simulink model "BrowarModel"  (R2024a)
settings: Solver=ode5  StartTime=0.0  StopTime=inf  FixedStep=0.1  RelTol=1e-3
undefined symbols (not defined in the file or in its folder): localhost, Matrikon, OI
libraries: opclib x24
(part 5 of 9)

== system BrowarModel/Kadz warzelna/Kadz warzelna/Model akumulacji ciepla w zbiorniku z ciecza ==
  Objetosc cieczy w zbiorniku : Inport
  Strumien odplywu cieczy : Inport  Port=2
  Strumien doplywu cieczy : Inport  Port=3
  Strumien cieplna dostepny : Inport  Port=4
  Strumien cieplo traconego : Inport  Port=5
  Temperatura strumien doplywu cieczy : Inport  Port=6
  1/gestosc cieczy : Gain  Gain=1/1000
  Cieplo : Integrator  LimitOutput=on  LowerSaturationLimit=0
  Cieplo parowania : Constant  Value=2257000
  Cieplo strumienia cieczy doplywajacej : Subsystem
  Cieplo strumienia cieczy odplywajacej : Subsystem
  "Cieplo wlasciwe " : Constant  Value=4189.9
  Display{,1..8} (9 alike) : Display
  Divide : Product  Inputs=/*
  Divide1 : Product  Inputs=*/
  Divide2 : Product  Inputs=*/
  "Dot " : DotProduct  OutDataTypeStr=Inherit: Inherit via internal rule
  Dot 1 : DotProduct  OutDataTypeStr=Inherit: Inherit via internal rule
  Gestosc cieczy : Gain  Gain=1000
  Saturation : Saturate  UpperLimit=inf  LowerLimit=0
  Sum{1..2,4..5} (4 alike) : Sum  Inputs=|+-
  Sum10 : Sum  Inputs=|++
  Sum3 : Sum  Inputs=|-+
  Sum7 : Sum  Inputs=|++
  Temperatura parowania : Constant  Value=100
  Zamiana C->K : Constant  Value=273.6
  Srumien cieczy odparowanej : Outport
  Srednia temperaturacie czy : Outport  Port=2
  Strumien ciepla odebrany : Outport  Port=3
  wires:
  Strumien cieplna dostepny/1 -> Strumien ciepla odebrany/1, Sum10/2  "J/s"
  Sum5/1 -> Sum4/1, Srednia temperaturacie czy/1, Display3/1
  Strumien doplywu cieczy/1 -> Cieplo strumienia cieczy doplywajacej/2(Strumien cieczy), Display6/1  "m3/s"
  Zamiana C->K/1 -> Sum5/2
  "Cieplo wlasciwe "/1 -> Divide1/2, Dot 1/2  "J/(kg*K)"
  Cieplo strumienia cieczy doplywajacej/1(Strumien ciepla) -> Sum3/2, Display1/1  "J/s"
  Temperatura strumien doplywu cieczy/1 -> Cieplo strumienia cieczy doplywajacej/1(Temperatura strumienia cieczy), Display8/1  "dec C"
  Divide1/1 -> Sum5/1, Cieplo strumienia cieczy odplywajacej/1(Temperatura strumienia cieczy)  "dec K"
  Divide/1 -> Divide1/1
  Cieplo/1 -> Divide/2, Display2/1  "J"
  Sum3/1 -> Sum1/1  "J/s"
  Strumien cieplo traconego/1 -> Sum1/2, Display7/1  "J/s"
  Sum1/1 -> Sum10/1  "J/s"
  Sum10/1 -> Sum2/1  "J/s"
  Temperatura parowania/1 -> Sum4/2  "dec C"
  Sum4/1 -> Saturation/1
  Saturation/1 -> Dot 1/1
  Dot 1/1 -> "Dot "/1
  "Dot "/1 -> Divide2/1, Sum2/2  "J/s"
  Sum2/1 -> Cieplo/1  "J/s"
  Cieplo strumienia cieczy odplywajacej/1(Strumien ciepla) -> Sum3/1, Display/1  "J/s"
  1/gestosc cieczy/1 -> Sum7/2, Srumien cieczy odparowanej/1  "m3/s"
  Divide2/1 -> 1/gestosc cieczy/1  "kg/s"
  Cieplo parowania/1 -> Divide2/2  "J/kg"
  Objetosc cieczy w zbiorniku/1 -> Gestosc cieczy/1  "m3"
  Gestosc cieczy/1 -> "Dot "/2, Divide/1, Display4/1  "kg"
  Sum7/1 -> Cieplo strumienia cieczy odplywajacej/2(Strumien cieczy)
  Strumien odplywu cieczy/1 -> Sum7/1, Display5/1  "m3/s"

== system BrowarModel/Kadz warzelna/Kadz warzelna/Model jakosci brzeczki wejsciowej ==
  note: Model jakosci brzeczki w zbiorniku
  Objetosc : Inport
  Przepelnienie : Inport  Port=2
  Doplyw brzeczki : Inport  Port=3
  Odplyw : Inport  Port=4
  Jakosc brzeczki : Inport  Port=5
  Divide1 : Product  Inputs=/*
  Jakosc brzeczki x objetosc : Integrator  LimitOutput=on  LowerSaturationLimit=0
  Product3 : Product  RndMeth=Zero
  Product4 : Product  RndMeth=Zero
  Product6 : Product  RndMeth=Zero
  Relational Operator : RelationalOperator  Operator=<  InputSameDT=off
  Sat : Constant
  Sum5 : Sum  Inputs=|+-
  Jakosc brzeczki zbiornika : Outport
  wires:
  Sum5/1 -> Jakosc brzeczki x objetosc/1
  Product4/1 -> Product3/2
  Sat/1 -> Relational Operator/2
  Jakosc brzeczki x objetosc/1 -> Divide1/2
  Divide1/1 -> Product6/1, Jakosc brzeczki zbiornika/1
  Product3/1 -> Sum5/1
  Relational Operator/1 -> Product3/1
  Product6/1 -> Sum5/2
  Objetosc/1 -> Divide1/1
  Doplyw brzeczki/1 -> Product4/1
  Odplyw/1 -> Product6/2
  Przepelnienie/1 -> Relational Operator/1
  Jakosc brzeczki/1 -> Product4/2

== system BrowarModel/Kadz warzelna/Kadz warzelna/Model jakosci warzenia ==
  note: Model jakosci warzenia
  Srednia temperatura : Inport
  Odplyw : Inport  Port=2
  Doplyw brzeczki : Inport  Port=3
  Doplyw chmielu : Inport  Port=4
  Constant : Constant  Value=48
  Display : Display
  Display1 : Display
  Divide : Product  Inputs=*/
  Divide1 : Product  Inputs=/*
  "Gotowanie " : Subsystem
  Jakosc mieszaniny : Lookup  InputValues=[0 0.001 0.00175 0.001875 0.002 0.002125 0.00225 0.003 0.005 0.0075]  Table=[0 0.2 0.5 1 1 1 0.5 0.2 0 0]  SaturateOnIntegerOverflow=off
  Objetosc brzeczka : Integrator  InitialCondition=0.001  LimitOutput=on  UpperSaturationLimit=48  LowerSaturationLimit=0.001
  Objetosc chmiel : Integrator  LimitOutput=on  UpperSaturationLimit=48  LowerSaturationLimit=0
  Odplyw brzeczka : DotProduct  OutDataTypeStr=Inherit: Inherit via internal rule
  Odplyw chmielu : DotProduct  OutDataTypeStr=Inherit: Inherit via internal rule
  Przepelnienie - brzeczka : DotProduct  OutDataTypeStr=Inherit: Inherit via internal rule
  Przepelnienie - chmiel : DotProduct  OutDataTypeStr=Inherit: Inherit via internal rule
  Relational Operator : RelationalOperator  Operator=<  InputSameDT=off
  Saturation : Saturate  UpperLimit=inf  LowerLimit=0
  Sum5 : Sum  Inputs=-+
  Sum6 : Sum  Inputs=+-
  Sum7 : Sum
  Jakosc : Outport
  wires:
  Sum6/1 -> Objetosc brzeczka/1
  Odplyw brzeczka/1 -> Sum6/2
  Objetosc chmiel/1 -> Sum7/1, Divide/1
  Objetosc brzeczka/1 -> Sum7/2, Divide1/2
  Sum7/1 -> Divide1/1, Divide/2, Relational Operator/1, "Gotowanie "/3(Objetosc mieszaniny)  "m3"
  Odplyw chmielu/1 -> Sum5/1
  Divide/1 -> Odplyw chmielu/1, Jakosc mieszaniny/1
  Divide1/1 -> Odplyw brzeczka/2
  Sum5/1 -> Objetosc chmiel/1
  Przepelnienie - chmiel/1 -> Sum5/2
  Przepelnienie - brzeczka/1 -> Sum6/1
  Relational Operator/1 -> Przepelnienie - chmiel/2, Przepelnienie - brzeczka/1
  Constant/1 -> Relational Operator/2
  Odplyw/1 -> Odplyw brzeczka/1, "Gotowanie "/4(Odplyw), Odplyw chmielu/2  "m3/s"
  "Gotowanie "/1(Jakosc) -> Saturation/1, Display1/1
  Jakosc mieszaniny/1 -> "Gotowanie "/2(Jakosc mieszaniny), Display/1  "[0,1]"
  Saturation/1 -> Jakosc/1
  Srednia temperatura/1 -> "Gotowanie "/1(Srednia temperatura)  "decC"
  Doplyw chmielu/1 -> Przepelnienie - chmiel/1  "m3/s"
  Doplyw brzeczki/1 -> Przepelnienie - brzeczka/2  "m3/s"

== system BrowarModel/Kadz warzelna/Kadz warzelna/Model ogrzewacza ==
  note: Ogrzewacz elektryczny
  note: Uszkodzenie ogrzewacza
  Sterowanie : Inport
  Spadek mocy : Inport  Port=2
  Booster : Product  RndMeth=Zero
  "Booster " : Subsystem
  Booster block : Subsystem
  Const : Constant  Value=100
  GUIMon : Gain
  Gain : Gain  Gain=1/100
  Gain1 : Gain  Gain=1/100
  Maksymalna moc : Constant  Value=10000000
  Product : Product  RndMeth=Zero
  Product1 : Product  RndMeth=Zero
  Quantizer : Quantizer  QuantizationInterval=20
  Sat ster : Saturate  UpperLimit=100  LowerLimit=0
  Sat uszk : Saturate  UpperLimit=100  LowerLimit=0
  Sat zero : Saturate  UpperLimit=inf  LowerLimit=0
  Sum1 : Sum  Inputs=|+-
  Sum2 : Sum  Inputs=|+-
  Transfer Fcn : TransferFcn  Denominator=[30 1]
  Transfer Fcn1 : TransferFcn  Denominator=[30 1]
  Zaklocenia : Subsystem
  Cieplo dostarczone : Outport
  wires:
  Sat ster/1 -> Quantizer/1
  Sterowanie/1 -> Sat ster/1
  Quantizer/1 -> GUIMon/1
  Gain/1 -> Product/1
  Zaklocenia/1(Out) -> Sum1/2
  Product/1 -> Transfer Fcn/1
  Transfer Fcn/1 -> Transfer Fcn1/1, "Booster "/1(In1)
  Sum1/1 -> Sat zero/1
  GUIMon/1 -> Gain/1
  Sat zero/1 -> Cieplo dostarczone/1
  Maksymalna moc/1 -> Product1/1
  Spadek mocy/1 -> Sat uszk/1
  Sat uszk/1 -> Sum2/2
  Sum2/1 -> Gain1/1
  Const/1 -> Sum2/1
  Gain1/1 -> Product1/2
  Product1/1 -> Booster/1
  Booster block/1(Out) -> Booster/2
  Booster/1 -> Product/2
  "Booster "/1(Out) -> Zaklocenia/1(In), Sum1/1
  Transfer Fcn1/1 -> "Booster "/2(In2)

== system BrowarModel/Kadz warzelna/Kadz warzelna/Model rozkladu temperatur ==
  Poziom : Inport
  Srednia temperatura : Inport  Port=2
  " Dot 1" : DotProduct  OutDataTypeStr=Inherit: Inherit via internal rule
  " Dot 2" : DotProduct  OutDataTypeStr=Inherit: Inherit via internal rule
  " Dot 3" : DotProduct  OutDataTypeStr=Inherit: Inherit via internal rule
  Divide2 : Product  Inputs=/*
  Divide3 : Product  Inputs=/*
  Divide4 : Product  Inputs=/*
  Model rozkladu temperatur : Subsystem
  Pozycja sensor dolny : Constant  Value=0.5
  Pozycja sensor gorny : Constant  Value=2.5
  Pozycja sensor srodkowy : Constant  Value=1.5
  Sensor dolny niezanuzony : RelationalOperator  Operator=<  InputSameDT=off
  Sensor gorny niezanuzony : RelationalOperator  Operator=<  InputSameDT=off
  Sensor srodkowy niezanuzony : RelationalOperator  Operator=<  InputSameDT=off
  Sum13 : Sum  Inputs=|+-
  Sum14 : Sum  Inputs=|+-
  Sum15 : Sum  Inputs=|+-
  Switch : Switch  Threshold=0.5  SaturateOnIntegerOverflow=off  InputSameDT=off
  Switch1 : Switch  Threshold=0.5  SaturateOnIntegerOverflow=off  InputSameDT=off
  Switch2 : Switch  Threshold=0.5  SaturateOnIntegerOverflow=off  InputSameDT=off
  "Temperatura pokojowa (deg C) " : Constant  Value=22
  Temperatura lustra zbiornika : Outport
  Sensor temperatury gorny : Outport  Port=2
  Sensor temperatury srodkowy : Outport  Port=3
  Sensor temperatury dolny : Outport  Port=4
  Temperatura przy dnie zbiornika : Outport  Port=5
  wires:
  Model rozkladu temperatur/1(Temperatura przy powierzchni) -> Temperatura lustra zbiornika/1
  Poziom/1 -> Divide4/1, Divide3/1, Divide2/1, Sensor dolny niezanuzony/1, Sensor srodkowy niezanuzony/1, Sensor gorny niezanuzony/1, Model rozkladu temperatur/1(Poziom)  "m"
  Switch2/1 -> Sensor temperatury dolny/1
  Switch/1 -> Sensor temperatury gorny/1
  " Dot 3"/1 -> Sum15/2
  Divide2/1 -> " Dot 3"/2
  Divide3/1 -> " Dot 2"/2
  " Dot 2"/1 -> Sum14/2
  " Dot 1"/1 -> Sum13/2
  Divide4/1 -> " Dot 1"/2
  Model rozkladu temperatur/2(Temperatura przy dnie) -> Sum15/1, Sum14/1, Sum13/1, Temperatura przy dnie zbiornika/1
  Sum15/1 -> Switch2/3
  Sum14/1 -> Switch1/3
  Sum13/1 -> Switch/3
  Switch1/1 -> Sensor temperatury srodkowy/1
  Sensor dolny niezanuzony/1 -> Switch2/2
  Sensor srodkowy niezanuzony/1 -> Switch1/2
  Sensor gorny niezanuzony/1 -> Switch/2
  Pozycja sensor dolny/1 -> Divide2/2, Sensor dolny niezanuzony/2
  Pozycja sensor srodkowy/1 -> Divide3/2, Sensor srodkowy niezanuzony/2
  Pozycja sensor gorny/1 -> Divide4/2, Sensor gorny niezanuzony/2
  "Temperatura pokojowa (deg C) "/1 -> Switch2/1, Switch1/1, Switch/1, Model rozkladu temperatur/2(Temperatura otoczenia)
  Model rozkladu temperatur/3(Gradient temperatury) -> " Dot 1"/1, " Dot 2"/1, " Dot 3"/1
  Srednia temperatura/1 -> Model rozkladu temperatur/3(Srednia temperatura)  "decC"

== system BrowarModel/Kadz warzelna/Kadz warzelna/Model utratu ciepla ==
  Poziom : Inport
  Pole podstawy zbiornika : Inport  Port=2
  Srednia temperatura : Inport  Port=3
  Temperatura lustra : Inport  Port=4
  Cieplo tracone przez pow. gorna : DotProduct  OutDataTypeStr=Inherit: Inherit via internal rule
  Cieplo tracone przez scianki : DotProduct  OutDataTypeStr=Inherit: Inherit via internal rule
  Pow ->obwod : Fcn  Expr=2*3.14*sqrt(u(1)/3.14)
  Pow styku scian bocznych : DotProduct  OutDataTypeStr=Inherit: Inherit via internal rule
  Saturation : Saturate  UpperLimit=inf  LowerLimit=0
  Sum11 : Sum  Inputs=|-+
  Sum12 : Sum  Inputs=|-+
  Sum2 : Sum
  "Temperatura pokojowa (deg C)  " : Constant  Value=22
  Wspolczynnik przenikania ciepla : Gain  Gain=950
  Wspolczynnik przenikania ciepla scian : Gain  Gain=450
  Strumien ciepla : Outport
  wires:
  Temperatura lustra/1 -> Sum12/2  "dec C"
  Sum2/1 -> Saturation/1
  Srednia temperatura/1 -> Sum11/2  "dec C"
  Pole podstawy zbiornika/1 -> Wspolczynnik przenikania ciepla/1, Pow ->obwod/1
  Poziom/1 -> Pow styku scian bocznych/1
  Sum11/1 -> Cieplo tracone przez scianki/2
  "Temperatura pokojowa (deg C)  "/1 -> Sum12/1, Sum11/1
  Cieplo tracone przez pow. gorna/1 -> Sum2/2
  Cieplo tracone przez scianki/1 -> Sum2/1
  Wspolczynnik przenikania ciepla scian/1 -> Cieplo tracone przez scianki/1
  Pow styku scian bocznych/1 -> Wspolczynnik przenikania ciepla scian/1  "m2"
  Pow ->obwod/1 -> Pow styku scian bocznych/2
  Sum12/1 -> Cieplo tracone przez pow. gorna/1
  Wspolczynnik przenikania ciepla/1 -> Cieplo tracone przez pow. gorna/2
  Saturation/1 -> Strumien ciepla/1  "J/s"

== system BrowarModel/Kadz warzelna/Kadz warzelna/Odplyw z kadzi ==
  note: Doplyw kadzi
  Sterowanie zaworu : Inport
  Przeciek zaworu : Inport  Port=2
  Dlawienie zaworu : Inport  Port=3
  Wyciek : Inport  Port=4
  Poziom w kadzi : Inport  Port=5
  Zalaczenie pompy : Inport  Port=6
  Sterowanie pompy : Inport  Port=7
  Uszkodzenie pompy : Inport  Port=8
  Charakterystyka pompy : Lookup  InputValues="[0\t125\t250\t375\t500\t625\t750\t875\t1000\t1125\t1250\t1375\t1500 1625]"  Table=|  SaturateOnIntegerOverflow=off
      | [0 50	125	178	220	250	270	288	300	310	315	320	323	327
      | ]
  Gain : Gain  Gain=1/100
  Obciazenie silnika : Gain  Gain=1/500
  Product : Product  RndMeth=Zero
  Product1 : Product  RndMeth=Zero
  Relay : Relay  OnOutputValue=0  OffOutputValue=1
  Relay1 : Relay
  Sat uszk : Saturate  UpperLimit=100  LowerLimit=0
  Silnik elektryczny : Subsystem
  "Sterowanie " : DotProduct  OutDataTypeStr=Inherit: Inherit via internal rule
  Straty pompy : Gain  Gain=50/0.15
  Sum : Sum  Inputs=|+-
  Sum1 : Sum  Inputs=|+-
  Wplyw stopnia wypelnienia kadzi : Lookup  InputValues=[-1, 0, 0.05, 1]  Table=[0, 0, 1,1]  SaturateOnIntegerOverflow=off
  Wplyw uszkodzenia : Product  RndMeth=Zero
  Zawor dyskretny : Subsystem
  Przeplyw_wyciek : Outport
  Przeplyw : Outport  Port=2
  Obroty : Outport  Port=3
  Prad silnika : Outport  Port=4
  Silnik Idle : Outport  Port=5
  Silnik Running : Outport  Port=6
  Silnik Alarm : Outport  Port=7
  wires:
  Wplyw stopnia wypelnienia kadzi/1 -> Product/1  "[0,1]"
  Zawor dyskretny/1(Przeplyw) -> Sum1/1, Straty pompy/1, Product1/1
  Dlawienie zaworu/1 -> Zawor dyskretny/4(Dlawienie)
  Poziom w kadzi/1 -> Wplyw stopnia wypelnienia kadzi/1  "m"
  Zalaczenie pompy/1 -> Relay1/1, Silnik elektryczny/1(Zalaczenie)
  Uszkodzenie pompy/1 -> Relay/1, Silnik elektryczny/4(Uszkodzenie)
  Relay/1 -> Wplyw uszkodzenia/2
  Silnik elektryczny/1(Obroty) -> Charakterystyka pompy/1, Obroty/1
  Wplyw uszkodzenia/1 -> Product/2
  Charakterystyka pompy/1 -> "Sterowanie "/2  "kPa"
  "Sterowanie "/1 -> Wplyw uszkodzenia/1
  Relay1/1 -> "Sterowanie "/1
  Product/1 -> Sum/1, Obciazenie silnika/1
  Sum/1 -> Zawor dyskretny/2(Cisnienie)
  Straty pompy/1 -> Sum/2
  Wyciek/1 -> Sat uszk/1
  Product1/1 -> Przeplyw_wyciek/1, Sum1/2
  Sum1/1 -> Przeplyw/1
  Sat uszk/1 -> Gain/1
  Przeciek zaworu/1 -> Zawor dyskretny/3(Przeciek)
  Sterowanie zaworu/1 -> Zawor dyskretny/1(Sterowanie)
  Gain/1 -> Product1/2
  Silnik elektryczny/2(Prad) -> Prad silnika/1
  Silnik elektryczny/3(Idle) -> Silnik Idle/1
  Silnik elektryczny/4(Running) -> Silnik Running/1
  Silnik elektryczny/5(Alarm) -> Silnik Alarm/1
  Sterowanie pompy/1 -> Silnik elektryczny/2(Zadane obroty)
  Obciazenie silnika/1 -> Silnik elektryczny/3(Obciazenie zew)

== system BrowarModel/Kadz warzelna/Kadz warzelna/Poziom zbiornika ==
  Objetosc : Inport
  Powierzchnia dna : Inport  Port=2
  1/powierzchnia : Product  Inputs=*/
  Pozycja sensora max (2.8 m) : Constant  Value=2.8
  Pozycja sensora min (0.2 m) : Constant  Value=.2
  Sensor max : RelationalOperator  InputSameDT=off
  Sensor min : RelationalOperator  InputSameDT=off
  Poziom  wysoki : Outport
  Poziom niski : Outport  Port=2
  Poziom : Outport  Port=3
  wires:
  Objetosc/1 -> 1/powierzchnia/1  "m3"
  Powierzchnia dna/1 -> 1/powierzchnia/2  "m2"
  Sensor min/1 -> Poziom niski/1
  Sensor max/1 -> Poziom  wysoki/1
  Pozycja sensora min (0.2 m)/1 -> Sensor min/2
  Pozycja sensora max (2.8 m)/1 -> Sensor max/2
  1/powierzchnia/1 -> Poziom/1, Sensor max/1, Sensor min/1  "m"

== system BrowarModel/Kadz warzelna/Kadz warzelna/Wyciek ==
  note: Kadz warzelna - wyciek
  Wyciek : Inport
  Poziom : Inport  Port=2
  Gain : Gain  Gain=1/3
  Math Function : Math  Operator=sqrt  SignedPower=on
  Max wyciek : Constant  Value=0.1
  Product : Product  RndMeth=Zero
  Product1 : Product  RndMeth=Zero
  Sat uszk (F>=0)1 : Saturate  UpperLimit=1  LowerLimit=0
  Strumien wycieku : Outport
  wires:
  Sat uszk (F>=0)1/1 -> Product/1
  Product1/1 -> Product/2
  Max wyciek/1 -> Product1/1  "m3/s"
  Math Function/1 -> Product1/2
  Gain/1 -> Math Function/1
  Poziom/1 -> Gain/1
  Wyciek/1 -> Sat uszk (F>=0)1/1
  Product/1 -> Strumien wycieku/1

== system BrowarModel/Kadz warzelna/LT401/Zaklocenia pomiarowe ==
  Product1 : Product  InputSameDT=on  RndMeth=Zero  SaturateOnIntegerOverflow=on  OutDataTypeStr=Inherit: Same as first input
  Product3 : Product  InputSameDT=on  RndMeth=Zero  SaturateOnIntegerOverflow=on  OutDataTypeStr=Inherit: Same as first input
  Random Number : RandomNumber  Variance=.5  Seed=4365624  SampleTime=0.1
  Transfer Fcn1 : TransferFcn  Denominator=[0.5 1]
  Transfer Fcn2 : TransferFcn  Denominator=[0.5 1]
  Zaklocenia pomiarowe : Constant  Value=ZakloceniaPom
  Out : Outport
  wires:
  Product1/1 -> Product3/2
  [ZaklPom] -> Product1/1
  Zaklocenia pomiarowe/1 -> Product1/2
  Transfer Fcn2/1 -> Out/1
  Transfer Fcn1/1 -> Transfer Fcn2/1
  Product3/1 -> Transfer Fcn1/1
  Random Number/1 -> Product3/1

== system BrowarModel/Kadz warzelna/ST404/Zaklocenia pomiarowe ==
  Product1 : Product  InputSameDT=on  RndMeth=Zero  SaturateOnIntegerOverflow=on  OutDataTypeStr=Inherit: Same as first input
  Product3 : Product  InputSameDT=on  RndMeth=Zero  SaturateOnIntegerOverflow=on  OutDataTypeStr=Inherit: Same as first input
  Random Number : RandomNumber  Variance=.5  Seed=4365624  SampleTime=0.1
  Transfer Fcn1 : TransferFcn  Denominator=[0.5 1]
  Transfer Fcn2 : TransferFcn  Denominator=[0.5 1]
  Zaklocenia pomiarowe : Constant  Value=ZakloceniaPom
  Out : Outport
  wires:
  Product1/1 -> Product3/2
  [ZaklPom] -> Product1/1
  Zaklocenia pomiarowe/1 -> Product1/2
  Transfer Fcn2/1 -> Out/1
  Transfer Fcn1/1 -> Transfer Fcn2/1
  Product3/1 -> Transfer Fcn1/1
  Random Number/1 -> Product3/1

== system BrowarModel/Kadz warzelna/TT402H/Zaklocenia pomiarowe ==
  Product1 : Product  InputSameDT=on  RndMeth=Zero  SaturateOnIntegerOverflow=on  OutDataTypeStr=Inherit: Same as first input
  Product3 : Product  InputSameDT=on  RndMeth=Zero  SaturateOnIntegerOverflow=on  OutDataTypeStr=Inherit: Same as first input
  Random Number : RandomNumber  Variance=.5  Seed=4365624  SampleTime=0.1
  Transfer Fcn1 : TransferFcn  Denominator=[0.5 1]
  Transfer Fcn2 : TransferFcn  Denominator=[0.5 1]
  Zaklocenia pomiarowe : Constant  Value=ZakloceniaPom
  Out : Outport
  wires:
  Random Number/1 -> Product3/1
  Product3/1 -> Transfer Fcn1/1
  Transfer Fcn1/1 -> Transfer Fcn2/1
  Transfer Fcn2/1 -> Out/1
  Zaklocenia pomiarowe/1 -> Product1/2
  [ZaklPom] -> Product1/1
  Product1/1 -> Product3/2

== system BrowarModel/Kadz warzelna/TT402L/Zaklocenia pomiarowe ==
  Product1 : Product  InputSameDT=on  RndMeth=Zero  SaturateOnIntegerOverflow=on  OutDataTypeStr=Inherit: Same as first input
  Product3 : Product  InputSameDT=on  RndMeth=Zero  SaturateOnIntegerOverflow=on  OutDataTypeStr=Inherit: Same as first input
  Random Number : RandomNumber  Variance=.5  Seed=4365624  SampleTime=0.1
  Transfer Fcn1 : TransferFcn  Denominator=[0.5 1]
  Transfer Fcn2 : TransferFcn  Denominator=[0.5 1]
  Zaklocenia pomiarowe : Constant  Value=ZakloceniaPom
  Out : Outport
  wires:
  Random Number/1 -> Product3/1
  Product3/1 -> Transfer Fcn1/1
  Transfer Fcn1/1 -> Transfer Fcn2/1
  Transfer Fcn2/1 -> Out/1
  Zaklocenia pomiarowe/1 -> Product1/2
  [ZaklPom] -> Product1/1
  Product1/1 -> Product3/2

== system BrowarModel/Kadz warzelna/TT402M/Zaklocenia pomiarowe ==
  Product1 : Product  InputSameDT=on  RndMeth=Zero  SaturateOnIntegerOverflow=on  OutDataTypeStr=Inherit: Same as first input
  Product3 : Product  InputSameDT=on  RndMeth=Zero  SaturateOnIntegerOverflow=on  OutDataTypeStr=Inherit: Same as first input
  Random Number : RandomNumber  Variance=.5  Seed=4365624  SampleTime=0.1
  Transfer Fcn1 : TransferFcn  Denominator=[0.5 1]
  Transfer Fcn2 : TransferFcn  Denominator=[0.5 1]
  Zaklocenia pomiarowe : Constant  Value=ZakloceniaPom
  Out : Outport
  wires:
  Product1/1 -> Product3/2
  [ZaklPom] -> Product1/1
  Zaklocenia pomiarowe/1 -> Product1/2
  Transfer Fcn2/1 -> Out/1
  Transfer Fcn1/1 -> Transfer Fcn2/1
  Product3/1 -> Transfer Fcn1/1
  Random Number/1 -> Product3/1

== system BrowarModel/Kadz zacierna/ET205/Zaklocenia pomiarowe ==
  Product1 : Product  InputSameDT=on  RndMeth=Zero  SaturateOnIntegerOverflow=on  OutDataTypeStr=Inherit: Same as first input
  Product3 : Product  InputSameDT=on  RndMeth=Zero  SaturateOnIntegerOverflow=on  OutDataTypeStr=Inherit: Same as first input
  Random Number : RandomNumber  Variance=.5  Seed=4365624  SampleTime=0.1
  Transfer Fcn1 : TransferFcn  Denominator=[0.5 1]
  Transfer Fcn2 : TransferFcn  Denominator=[0.5 1]
  Zaklocenia pomiarowe : Constant  Value=ZakloceniaPom
  Out : Outport
  wires:
  Random Number/1 -> Product3/1
  Product3/1 -> Transfer Fcn1/1
  Transfer Fcn1/1 -> Transfer Fcn2/1
  Transfer Fcn2/1 -> Out/1
  Zaklocenia pomiarowe/1 -> Product1/2
  [ZaklPom] -> Product1/1
  Product1/1 -> Product3/2

== system BrowarModel/Kadz zacierna/FT201/Zaklocenia pomiarowe ==
  Product1 : Product  InputSameDT=on  RndMeth=Zero  SaturateOnIntegerOverflow=on  OutDataTypeStr=Inherit: Same as first input
  Product3 : Product  InputSameDT=on  RndMeth=Zero  SaturateOnIntegerOverflow=on  OutDataTypeStr=Inherit: Same as first input
  Random Number : RandomNumber  Variance=.5  Seed=4365624  SampleTime=0.1
  Transfer Fcn1 : TransferFcn  Denominator=[0.5 1]
  Transfer Fcn2 : TransferFcn  Denominator=[0.5 1]
  Zaklocenia pomiarowe : Constant  Value=ZakloceniaPom
  Out : Outport
  wires:
  Random Number/1 -> Product3/1
  Product3/1 -> Transfer Fcn1/1
  Transfer Fcn1/1 -> Transfer Fcn2/1
  Transfer Fcn2/1 -> Out/1
  Zaklocenia pomiarowe/1 -> Product1/2
  [ZaklPom] -> Product1/1
  Product1/1 -> Product3/2

== system BrowarModel/Kadz zacierna/Kadz zacierna/Kadz zacierna ==
  note: Kadz
  Doplyw wody : Inport
  Temperatura doplywu wody : Inport  Port=2
  Doplyw sruty : Inport  Port=3
  Temperatura doplywu sruty : Inport  Port=4
  Odplyw : Inport  Port=5
  Dostepny strumien ciepla : Inport  Port=6
  Obroty mieszadla : Inport  Port=7
  Wyciek : Inport  Port=8
  Gain : Gain  Gain=1/1.5
  Math Function : Math  Operator=sqrt  SignedPower=on
  Max wyciek : Constant  Value=0.1
  Model akumulacji ciepla w zbiorniku z ciecza : Subsystem
  Model jakosci zacieru : Subsystem
  Model rozkladu temperatur : Subsystem
  Model utratu ciepla : Subsystem
  Objetosc : Integrator  InitialCondition=0.001  LimitOutput=on  UpperSaturationLimit=48  LowerSaturationLimit=0.001  ShowSaturationPort=on
  Powierzchnia dna m2 : Constant  Value=32
  Poziom zbiornika : Subsystem
  Product : Product  RndMeth=Zero
  Product1 : Product  RndMeth=Zero
  Sat doplyw (F>=0) : Saturate  UpperLimit=inf  LowerLimit=0
  Sat uszk (F>=0)1 : Saturate  UpperLimit=1  LowerLimit=0
  Saturation : Saturate  UpperLimit=inf  LowerLimit=0
  Sum1 : Sum  Inputs=|+-
  Sum2 : Sum  Inputs=|+-
  Sum3 : Sum  Inputs=|++
  Sum4 : Sum  Inputs=|++
  Poziom : Outport
  Poziom wysoki : Outport  Port=2
  Poziom niski : Outport  Port=3
  Temperatura sensor gorny : Outport  Port=4
  Temperatura sensor srodkowy : Outport  Port=5
  Temperatura sensor dolny : Outport  Port=6
  Temperatura dna : Outport  Port=7
  Jakosc zacieru : Outport  Port=8
  Temperatura srednia : Outport  Port=9
  wires:
  Temperatura doplywu wody/1 -> Model akumulacji ciepla w zbiorniku z ciecza/6(Temperatura strumien doplywu wody)
  Model akumulacji ciepla w zbiorniku z ciecza/1(Srumien cieczy odparowanej) -> Sum2/2  "m3/s"
  Sum1/1 -> Sum2/1
  Sum2/1 -> Objetosc/1
  Poziom zbiornika/3(Poziom) -> Poziom/1, Model utratu ciepla/1(Poziom), Model rozkladu temperatur/1(Poziom), Gain/1
  Objetosc/1 -> Poziom zbiornika/1(Objetosc), Model akumulacji ciepla w zbiorniku z ciecza/1(Objetosc cieczy w zbiorniku)  "m3"
  Poziom zbiornika/1(Poziom  wysoki) -> Poziom wysoki/1
  Poziom zbiornika/2(Poziom niski) -> Poziom niski/1
  Powierzchnia dna m2/1 -> Poziom zbiornika/2(Powierzchnia dna), Model utratu ciepla/2(Pole podstawy zbiornika)  "m2"
  Model akumulacji ciepla w zbiorniku z ciecza/2(Srednia temperaturacie czy) -> Model utratu ciepla/3(Srednia temperatura), Model rozkladu temperatur/2(Srednia temperatura), Model jakosci zacieru/1(Srednia temperatura), Temperatura srednia/1
  Model utratu ciepla/1(Strumien ciepla) -> Model akumulacji ciepla w zbiorniku z ciecza/9(Strumien cieplo traconego)
  Model rozkladu temperatur/1(Temperatura lustra zbiornika) -> Model utratu ciepla/4(Temperatura lustra)  "dec C"
  Doplyw sruty/1 -> Sat doplyw (F>=0)/1
  Model rozkladu temperatur/2(Sensor temperatury gorny) -> Temperatura sensor gorny/1
  Model rozkladu temperatur/3(Sensor temperatury srodkowy) -> Temperatura sensor srodkowy/1
  Model rozkladu temperatur/4(Sensor temperatury dolny) -> Temperatura sensor dolny/1
  Obroty mieszadla/1 -> Model rozkladu temperatur/3(Obroty mieszadla), Model jakosci zacieru/5(Obroty mieszadla)
  Dostepny strumien ciepla/1 -> Model akumulacji ciepla w zbiorniku z ciecza/8(Strumien cieplna dostepny)  "J/s"
  Model rozkladu temperatur/5(Temperatura przy dnie zbiornika) -> Temperatura dna/1
  Sat doplyw (F>=0)/1 -> Sum3/1, Model akumulacji ciepla w zbiorniku z ciecza/5(Strumien sruty), Model jakosci zacieru/4(Doplyw srutu)  "m3/s"
  Sum3/1 -> Sum1/1
  Doplyw wody/1 -> Sum3/2, Model akumulacji ciepla w zbiorniku z ciecza/4(Strumien doplywu wody), Model jakosci zacieru/3(Doplyw wody)  "m3/h"
  Temperatura doplywu sruty/1 -> Model akumulacji ciepla w zbiorniku z ciecza/7(Temperatura strumien doplywu sruty)
  Sum4/1 -> Model akumulacji ciepla w zbiorniku z ciecza/3(Strumien odplywu cieczy), Model jakosci zacieru/2(Odplyw), Sum1/2
  Odplyw/1 -> Saturation/1  "m3/h"
  Wyciek/1 -> Sat uszk (F>=0)1/1
  Product/1 -> Sum4/2
  Sat uszk (F>=0)1/1 -> Product/1
  Model jakosci zacieru/1(Jakosc) -> Jakosc zacieru/1
  Product1/1 -> Product/2
  Max wyciek/1 -> Product1/1  "m3/s"
  Math Function/1 -> Product1/2
  Gain/1 -> Math Function/1
  Objetosc/2 -> Model akumulacji ciepla w zbiorniku z ciecza/2(Przepelnienie)
  Saturation/1 -> Sum4/1

== system BrowarModel/Kadz zacierna/Kadz zacierna/Model mieszadla ==
  note: Model mieszadla
  note: Uszkodzenie:
      | Poslizg przekladni
  Poziom : Inport
  Obroty : Inport  Port=2
  Poslizg przekladni : Inport  Port=3
  " Gain" : Gain  Gain=1/4
  " Gain1" : Gain  Gain=1/100
  " Redukcja obrotow" : Gain  Gain=1/720
  Constant : Constant  Value=100
  Dot : DotProduct  OutDataTypeStr=Inherit: Inherit via internal rule
  Dot Product : DotProduct  OutDataTypeStr=Inherit: Inherit via internal rule
  Math Function : Math  Operator=square  SignedPower=on
  Sat FS : Saturate  UpperLimit=1  LowerLimit=0
  Sat uszkodzenia [0,100] : Saturate  UpperLimit=100  LowerLimit=0
  Sum1 : Sum  Inputs=|-+
  Wplyw stopnia wypelnienia na obciazenie : Lookup  InputValues=[0,0.3,1,2]  Table=[0.1,0.1,1,1]  SaturateOnIntegerOverflow=off
  Obroty zredukowane : Outport
  Obciazenie : Outport  Port=2
  wires:
  Sat FS/1 -> Obciazenie/1
  Dot Product/1 -> Sat FS/1
  Wplyw stopnia wypelnienia na obciazenie/1 -> Dot Product/2
  " Gain"/1 -> Dot Product/1
  Math Function/1 -> " Gain"/1
  Poziom/1 -> Wplyw stopnia wypelnienia na obciazenie/1
  Obroty/1 -> " Redukcja obrotow"/1  "obr/min"
  Poslizg przekladni/1 -> Sat uszkodzenia [0,100]/1  "[0,100]"
  Sat uszkodzenia [0,100]/1 -> Sum1/1
  Sum1/1 -> " Gain1"/1
  Constant/1 -> Sum1/2
  " Redukcja obrotow"/1 -> Dot/2  "obr/min"
  Dot/1 -> Obroty zredukowane/1, Math Function/1
  " Gain1"/1 -> Dot/1

== system BrowarModel/Kadz zacierna/Kadz zacierna/Model ogrzewacza ==
  note: Ogrzewacz elektryczny
  note: Uszkodzenie ogrzewacza
  Sterowanie : Inport
  Spadek mocy : Inport  Port=2
  Booster : Product  RndMeth=Zero
  "Booster " : Subsystem
  Booster block : Subsystem
  Const : Constant  Value=100
  GUIMon : Gain
  Gain : Gain  Gain=1/100
  Gain1 : Gain  Gain=1/100
  Maksymalna moc : Constant  Value=10000000
  Product : Product  RndMeth=Zero
  Product1 : Product  RndMeth=Zero
  Quantizer : Quantizer  QuantizationInterval=20
  Sat ster : Saturate  UpperLimit=100  LowerLimit=0
  Sat uszk : Saturate  UpperLimit=100  LowerLimit=0
  Sat zero : Saturate  UpperLimit=inf  LowerLimit=0
  Sum1 : Sum  Inputs=|+-
  Sum2 : Sum  Inputs=|+-
  Transfer Fcn : TransferFcn  Denominator=[30 1]
  Transfer Fcn1 : TransferFcn  Denominator=[30 1]
  Zaklocenia : Subsystem
  Cieplo dostarczone : Outport
  wires:
  Sat ster/1 -> Quantizer/1
  Sterowanie/1 -> Sat ster/1
  Quantizer/1 -> GUIMon/1
  Gain/1 -> Product/1
  Zaklocenia/1(Out) -> Sum1/2
  Product/1 -> Transfer Fcn/1
  Transfer Fcn/1 -> Transfer Fcn1/1, "Booster "/1(In1)
  Sum1/1 -> Sat zero/1
  GUIMon/1 -> Gain/1
  Sat zero/1 -> Cieplo dostarczone/1
  Maksymalna moc/1 -> Product1/1
  Spadek mocy/1 -> Sat uszk/1
  Sat uszk/1 -> Sum2/2
  Sum2/1 -> Gain1/1
  Const/1 -> Sum2/1
  Gain1/1 -> Product1/2
  Product1/1 -> Booster/1
  Booster block/1(Out) -> Booster/2
  Booster/1 -> Product/2
  "Booster "/1(Out) -> Zaklocenia/1(In), Sum1/1
  Transfer Fcn1/1 -> "Booster "/2(In2)

== system BrowarModel/Kadz zacierna/Kadz zacierna/Silnik elektryczny ==
  note: Silnik elektryczny
  note: Uszkodzenie silnika
  Zalaczenie : Inport
  Zadane obroty : Inport  Port=2
  Obciazenie zew : Inport  Port=3
  Uszkodzenie : Inport  Port=4
  Abs : Abs  SaturateOnIntegerOverflow=off
  Add : Sum
  Add1 : Sum  Inputs=+-
  Const : Constant
  Gain : Gain
  "Hz -> obr/min" : Gain  Gain=60/2
  Inercja mechaniczna : TransferFcn  Denominator=[1 1]
  Poslizg : DotProduct  OutDataTypeStr=Inherit: Inherit via internal rule
  Poslizg jalowy : Constant  Value=0.04
  Poslizg od obciazenia : Gain  Gain=0.05
  Prad jalowy : Gain  Gain=0.5
  Prad nominalny (10A) : Constant  Value=10
  Relay : Relay  OnOutputValue=0  OffOutputValue=1
  Saturation [0,1] : Saturate  UpperLimit=1  LowerLimit=0
  "Saturation [0,1] " : Saturate  UpperLimit=1  LowerLimit=0
  Stan : Subsystem
  Sterowanie : Subsystem
  Sterownik : Subsystem
  Sum : Sum  Inputs=|+-
  Sum1 : Sum  Inputs=|++
  Sum2 : Sum  Inputs=|+-
  Sum3 : Sum  Inputs=|++
  Wplyw uszkodzenia : DotProduct  OutDataTypeStr=Inherit: Inherit via internal rule
  Wplyw obciazenia : DotProduct  OutDataTypeStr=Inherit: Inherit via internal rule
  Wplyw obrotow : DotProduct  OutDataTypeStr=Inherit: Inherit via internal rule
  Zaklocenia : Subsystem
  Zalaczony : DotProduct  OutDataTypeStr=Inherit: Inherit via internal rule
  "obr/min -> FS  " : Gain  Gain=1/1500
  "obr/min -> Hz" : Gain  Gain=1/60*2
  Obroty : Outport
  Prad : Outport  Port=2
  Idle : Outport  Port=3
  Running : Outport  Port=4
  Alarm : Outport  Port=5
  wires:
  Inercja mechaniczna/1 -> Obroty/1, Poslizg/1, Add1/2, "obr/min -> Hz"/1
  Sum/1 -> Inercja mechaniczna/1
  "Hz -> obr/min"/1 -> Sum2/1, Zaklocenia/1(In)  "[obr/min]"
  Poslizg/1 -> Sum/2
  Sum3/1 -> Poslizg/2
  Poslizg od obciazenia/1 -> Sum3/1
  Obciazenie zew/1 -> Saturation [0,1]/1  "FS"
  Poslizg jalowy/1 -> Sum3/2
  Prad nominalny (10A)/1 -> Prad jalowy/1  "A"
  Prad jalowy/1 -> Sum1/2, Wplyw obciazenia/2
  Wplyw obciazenia/1 -> Sum1/1
  Abs/1 -> Wplyw obciazenia/1  "FS"
  Const/1 -> Wplyw obrotow/1
  "obr/min -> Hz"/1 -> Sterownik/1(PV)
  Saturation [0,1]/1 -> Add/2
  Add/1 -> Poslizg od obciazenia/1, Abs/1  "FS"
  Add1/1 -> "obr/min -> FS  "/1
  "obr/min -> FS  "/1 -> Gain/1
  "Saturation [0,1] "/1 -> Add/1
  Zalaczenie/1 -> Sterowanie/2(Zalaczenie), Stan/1(Zalaczony)
  Sterowanie/1(Sterowanie) -> Sterownik/2(SP)
  Gain/1 -> "Saturation [0,1] "/1
  Uszkodzenie/1 -> Relay/1
  Sterownik/1(CV) -> Wplyw uszkodzenia/1
  Relay/1 -> Wplyw uszkodzenia/2, Stan/2(Zdatny)
  Wplyw uszkodzenia/1 -> "Hz -> obr/min"/1
  Wplyw obrotow/1 -> Prad/1  "A"
  Sum1/1 -> Zalaczony/1  "A"
  Zalaczony/1 -> Wplyw obrotow/2
  Zadane obroty/1 -> Sterowanie/1(Zadane obroty)
  Stan/1(Idle) -> Idle/1
  Stan/2(Running) -> Running/1, Zalaczony/2
  Stan/3(Alarm) -> Alarm/1
  Sum2/1 -> Add1/1, Sum/1
  Zaklocenia/1(Out) -> Sum2/2

== system BrowarModel/Kadz zacierna/Kadz zacierna/Zawor doplywu wody ==
  note: Zawor doplywu slodu
  note: Uszkodzenie:
      | Brak materialu
  note: Uszkodzenie:
      | Dlawienie przeplywu w zaworze
  note: Uszkodzenie:
      | Przeciek wewnetrzny w zaworze
  note: Uszkodzenie:
      | Wyciek zewnetrzny w zaworze
  Sterowanie : Inport
  Dlawienie : Inport  Port=2
  Przeciek : Inport  Port=3
  Wyciek : Inport  Port=4
  Brak : Inport  Port=5
  Booster : Product  RndMeth=Zero
  Booster block : Subsystem
  Const : Constant  Value=100
  Const1 : Constant  Value=100
  Const2 : Constant  Value=100
  Dead Zone : DeadZone  LowerValue=-inf  UpperValue=0.0002
  GUIMon : Gain
  Gain : Gain  Gain=1/100
  Gain1 : Gain  Gain=1/100
  Gain2 : Gain  Gain=1/100
  Integer Delay : Delay  DelayLength=15
  Napelnianie m3/s : Gain  Gain=Fmax/100
  Product : Product  RndMeth=Zero
  Product1 : Product  RndMeth=Zero
  Product2 : Product  RndMeth=Zero
  Relay : Relay  OnOutputValue=100
  Sat (0-100) : Saturate  UpperLimit=100  LowerLimit=0
  Sat dlawienie (0-100) : Saturate  UpperLimit=100  LowerLimit=0
  Sat przecieku (0-100) : Saturate  UpperLimit=100  LowerLimit=0
  Sat uszk (0-100) : Saturate  UpperLimit=100  LowerLimit=0
  Sat wyciek (0-100) : Saturate  UpperLimit=100  LowerLimit=0
  Sum : Sum  Inputs=|+-
  Sum1 : Sum  Inputs=|++
  Sum2 : Sum  Inputs=|+-
  Sum3 : Sum  Inputs=|+-
  Sum5 : Sum  Inputs=|++
  Transfer Fcn : TransferFcn  Denominator=[1 1]
  Zaklocenia : Subsystem
  Przeplyw : Outport
  wires:
  Product/1 -> Transfer Fcn/1  "m3/s"
  Const/1 -> Sum/1
  Sat dlawienie (0-100)/1 -> Sum/2
  Sum/1 -> Gain/1
  Transfer Fcn/1 -> Integer Delay/1  "m3/s"
  Sterowanie/1 -> Relay/1
  Dlawienie/1 -> Sat dlawienie (0-100)/1  "[0,100]"
  Sat (0-100)/1 -> Napelnianie m3/s/1
  Sum1/1 -> Sat (0-100)/1
  Relay/1 -> GUIMon/1
  Przeciek/1 -> Sat przecieku (0-100)/1
  Sat przecieku (0-100)/1 -> Sum1/2
  Wyciek/1 -> Sat wyciek (0-100)/1
  Const1/1 -> Sum2/1
  Sat wyciek (0-100)/1 -> Sum2/2
  Integer Delay/1 -> Product1/1  "m3/s"
  Product1/1 -> Dead Zone/1
  Sum2/1 -> Gain1/1
  Gain1/1 -> Product1/2
  Product2/1 -> Sum1/1
  GUIMon/1 -> Product2/2
  Brak/1 -> Sat uszk (0-100)/1
  Const2/1 -> Sum3/1
  Sat uszk (0-100)/1 -> Sum3/2
  Sum3/1 -> Gain2/1
  Sum5/1 -> Product/2
  Gain/1 -> Product/1
  Zaklocenia/1(Out) -> Sum5/2
  Gain2/1 -> Product2/1
  Napelnianie m3/s/1 -> Booster/1
  Booster/1 -> Sum5/1, Zaklocenia/1(In)
  Booster block/1(Out) -> Booster/2
  Dead Zone/1 -> Przeplyw/1

== system BrowarModel/Kadz zacierna/LT202/Zaklocenia pomiarowe ==
  Product1 : Product  InputSameDT=on  RndMeth=Zero  SaturateOnIntegerOverflow=on  OutDataTypeStr=Inherit: Same as first input
  Product3 : Product  InputSameDT=on  RndMeth=Zero  SaturateOnIntegerOverflow=on  OutDataTypeStr=Inherit: Same as first input
  Random Number : RandomNumber  Variance=.5  Seed=4365624  SampleTime=0.1
  Transfer Fcn1 : TransferFcn  Denominator=[0.5 1]
  Transfer Fcn2 : TransferFcn  Denominator=[0.5 1]
  Zaklocenia pomiarowe : Constant  Value=ZakloceniaPom
  Out : Outport
  wires:
  Product1/1 -> Product3/2
  [ZaklPom] -> Product1/1
  Zaklocenia pomiarowe/1 -> Product1/2
  Transfer Fcn2/1 -> Out/1
  Transfer Fcn1/1 -> Transfer Fcn2/1
  Product3/1 -> Transfer Fcn1/1
  Random Number/1 -> Product3/1

== system BrowarModel/Kadz zacierna/QT204/Zaklocenia ==
  note: Zaklocenia procesowe
  In : Inport
  Product3 : Product  InputSameDT=on  RndMeth=Zero  SaturateOnIntegerOverflow=on  OutDataTypeStr=Inherit: Same as first input
  Product4 : Product  InputSameDT=on  RndMeth=Zero  SaturateOnIntegerOverflow=on  OutDataTypeStr=Inherit: Same as first input
  Random Number : RandomNumber  Variance=0.1  Seed=4365624  SampleTime=0.1
  Transfer Fcn1 : TransferFcn  Denominator=[0.1 1]
  Out : Outport
  wires:
  [ZaklProc] -> Product3/2
  Random Number/1 -> Product3/1
  Product3/1 -> Transfer Fcn1/1
  Transfer Fcn1/1 -> Product4/2
  In/1 -> Product4/1
  Product4/1 -> Out/1

== system BrowarModel/Kadz zacierna/ST205/Zaklocenia pomiarowe ==
  Product1 : Product  InputSameDT=on  RndMeth=Zero  SaturateOnIntegerOverflow=on  OutDataTypeStr=Inherit: Same as first input
  Product3 : Product  InputSameDT=on  RndMeth=Zero  SaturateOnIntegerOverflow=on  OutDataTypeStr=Inherit: Same as first input
  Random Number : RandomNumber  Variance=.5  Seed=4365624  SampleTime=0.1
  Transfer Fcn1 : TransferFcn  Denominator=[0.5 1]
  Transfer Fcn2 : TransferFcn  Denominator=[0.5 1]
  Zaklocenia pomiarowe : Constant  Value=ZakloceniaPom
  Out : Outport
  wires:
  Product1/1 -> Product3/2
  [ZaklPom] -> Product1/1
  Zaklocenia pomiarowe/1 -> Product1/2
  Transfer Fcn2/1 -> Out/1
  Transfer Fcn1/1 -> Transfer Fcn2/1
  Product3/1 -> Transfer Fcn1/1
  Random Number/1 -> Product3/1

== system BrowarModel/Kadz zacierna/TT203H/Zaklocenia pomiarowe ==
  Product1 : Product  InputSameDT=on  RndMeth=Zero  SaturateOnIntegerOverflow=on  OutDataTypeStr=Inherit: Same as first input
  Product3 : Product  InputSameDT=on  RndMeth=Zero  SaturateOnIntegerOverflow=on  OutDataTypeStr=Inherit: Same as first input
  Random Number : RandomNumber  Variance=.5  Seed=4365624  SampleTime=0.1
  Transfer Fcn1 : TransferFcn  Denominator=[0.5 1]
  Transfer Fcn2 : TransferFcn  Denominator=[0.5 1]
  Zaklocenia pomiarowe : Constant  Value=ZakloceniaPom
  Out : Outport
  wires:
  Random Number/1 -> Product3/1
  Product3/1 -> Transfer Fcn1/1
  Transfer Fcn1/1 -> Transfer Fcn2/1
  Transfer Fcn2/1 -> Out/1
  Zaklocenia pomiarowe/1 -> Product1/2
  [ZaklPom] -> Product1/1
  Product1/1 -> Product3/2

== system BrowarModel/Kadz zacierna/TT203L/Zaklocenia pomiarowe ==
  Product1 : Product  InputSameDT=on  RndMeth=Zero  SaturateOnIntegerOverflow=on  OutDataTypeStr=Inherit: Same as first input
  Product3 : Product  InputSameDT=on  RndMeth=Zero  SaturateOnIntegerOverflow=on  OutDataTypeStr=Inherit: Same as first input
  Random Number : RandomNumber  Variance=.5  Seed=4365624  SampleTime=0.1
  Transfer Fcn1 : TransferFcn  Denominator=[0.5 1]
  Transfer Fcn2 : TransferFcn  Denominator=[0.5 1]
  Zaklocenia pomiarowe : Constant  Value=ZakloceniaPom
  Out : Outport
  wires:
  Random Number/1 -> Product3/1
  Product3/1 -> Transfer Fcn1/1
  Transfer Fcn1/1 -> Transfer Fcn2/1
  Transfer Fcn2/1 -> Out/1
  Zaklocenia pomiarowe/1 -> Product1/2
  [ZaklPom] -> Product1/1
  Product1/1 -> Product3/2

== system BrowarModel/Kadz zacierna/TT203M/Zaklocenia pomiarowe ==
  Product1 : Product  InputSameDT=on  RndMeth=Zero  SaturateOnIntegerOverflow=on  OutDataTypeStr=Inherit: Same as first input
  Product3 : Product  InputSameDT=on  RndMeth=Zero  SaturateOnIntegerOverflow=on  OutDataTypeStr=Inherit: Same as first input
  Random Number : RandomNumber  Variance=.5  Seed=4365624  SampleTime=0.1
  Transfer Fcn1 : TransferFcn  Denominator=[0.5 1]
  Transfer Fcn2 : TransferFcn  Denominator=[0.5 1]
  Zaklocenia pomiarowe : Constant  Value=ZakloceniaPom
  Out : Outport
  wires:
  Product1/1 -> Product3/2
  [ZaklPom] -> Product1/1
  Zaklocenia pomiarowe/1 -> Product1/2
  Transfer Fcn2/1 -> Out/1
  Transfer Fcn1/1 -> Transfer Fcn2/1
  Product3/1 -> Transfer Fcn1/1
  Random Number/1 -> Product3/1

== system BrowarModel/Mlyn browarniany/ET103/Zaklocenia pomiarowe ==
  Product1 : Product  InputSameDT=on  RndMeth=Zero  SaturateOnIntegerOverflow=on  OutDataTypeStr=Inherit: Same as first input
  Product3 : Product  InputSameDT=on  RndMeth=Zero  SaturateOnIntegerOverflow=on  OutDataTypeStr=Inherit: Same as first input
  Random Number : RandomNumber  Variance=.5  Seed=4365624  SampleTime=0.1
  Transfer Fcn1 : TransferFcn  Denominator=[0.5 1]
  Transfer Fcn2 : TransferFcn  Denominator=[0.5 1]
  Zaklocenia pomiarowe : Constant  Value=ZakloceniaPom
  Out : Outport
  wires:
  Random Number/1 -> Product3/1
  Product3/1 -> Transfer Fcn1/1
  Transfer Fcn1/1 -> Transfer Fcn2/1
  Transfer Fcn2/1 -> Out/1
  Zaklocenia pomiarowe/1 -> Product1/2
  [ZaklPom] -> Product1/1
  Product1/1 -> Product3/2

== system BrowarModel/Mlyn browarniany/ET105/Zaklocenia pomiarowe ==
  Product1 : Product  InputSameDT=on  RndMeth=Zero  SaturateOnIntegerOverflow=on  OutDataTypeStr=Inherit: Same as first input
  Product3 : Product  InputSameDT=on  RndMeth=Zero  SaturateOnIntegerOverflow=on  OutDataTypeStr=Inherit: Same as first input
  Random Number : RandomNumber  Variance=.5  Seed=4365624  SampleTime=0.1
  Transfer Fcn1 : TransferFcn  Denominator=[0.5 1]
  Transfer Fcn2 : TransferFcn  Denominator=[0.5 1]
  Zaklocenia pomiarowe : Constant  Value=ZakloceniaPom
  Out : Outport
  wires:
  Product1/1 -> Product3/2
  [ZaklPom] -> Product1/1
  Zaklocenia pomiarowe/1 -> Product1/2
  Transfer Fcn2/1 -> Out/1
  Transfer Fcn1/1 -> Transfer Fcn2/1
  Product3/1 -> Transfer Fcn1/1
  Random Number/1 -> Product3/1

== system BrowarModel/Mlyn browarniany/FT105/Zaklocenia pomiarowe ==
  Product1 : Product  InputSameDT=on  RndMeth=Zero  SaturateOnIntegerOverflow=on  OutDataTypeStr=Inherit: Same as first input
  Product3 : Product  InputSameDT=on  RndMeth=Zero  SaturateOnIntegerOverflow=on  OutDataTypeStr=Inherit: Same as first input
  Random Number : RandomNumber  Variance=.5  Seed=4365624  SampleTime=0.1
  Transfer Fcn1 : TransferFcn  Denominator=[0.5 1]
  Transfer Fcn2 : TransferFcn  Denominator=[0.5 1]
  Zaklocenia pomiarowe : Constant  Value=ZakloceniaPom
  Out : Outport
  wires:
  Product1/1 -> Product3/2
  [ZaklPom] -> Product1/1
  Zaklocenia pomiarowe/1 -> Product1/2
  Transfer Fcn2/1 -> Out/1
  Transfer Fcn1/1 -> Transfer Fcn2/1
  Product3/1 -> Transfer Fcn1/1
  Random Number/1 -> Product3/1

== system BrowarModel/Mlyn browarniany/LT102/Zaklocenia pomiarowe ==
  Product1 : Product  InputSameDT=on  RndMeth=Zero  SaturateOnIntegerOverflow=on  OutDataTypeStr=Inherit: Same as first input
  Product3 : Product  InputSameDT=on  RndMeth=Zero  SaturateOnIntegerOverflow=on  OutDataTypeStr=Inherit: Same as first input
  Random Number : RandomNumber  Variance=.5  Seed=4365624  SampleTime=0.1
  Transfer Fcn1 : TransferFcn  Denominator=[0.5 1]
  Transfer Fcn2 : TransferFcn  Denominator=[0.5 1]
  Zaklocenia pomiarowe : Constant  Value=ZakloceniaPom
  Out : Outport
  wires:
  Product1/1 -> Product3/2
  [ZaklPom] -> Product1/1
  Zaklocenia pomiarowe/1 -> Product1/2
  Transfer Fcn2/1 -> Out/1
  Transfer Fcn1/1 -> Transfer Fcn2/1
  Product3/1 -> Transfer Fcn1/1
  Random Number/1 -> Product3/1

== system BrowarModel/Mlyn browarniany/Mlyn browarniany/Dozownik mlyna ==
  note: Dozownik mlyna
  Zalaczenie silnika : Inport
  "Zadane obroty silnika " : Inport  Port=2
  Poziom zasobnika : Inport  Port=3
  Wyplnienie komory : Inport  Port=4
  Zanieczyszczenie lopatek : Inport  Port=5
  Blokada przeplywu : Inport  Port=6
  Przeciek w dozowniku : Inport  Port=7
  "Poslizg przekladni " : Inport  Port=8
  Uszkodzenie lozyska : Inport  Port=9
  Uszkodzenie silnika : Inport  Port=10
  Dozownik turbinowy : Subsystem
  Silnik elektryczny : Subsystem
  Przeplyw : Outport
  Temperatura lozyska : Outport  Port=2
  Obroty silnika : Outport  Port=3
  Prad silnika : Outport  Port=4
  Silnik Idle : Outport  Port=5
  Silnik Running : Outport  Port=6
  Silnik Alarm : Outport  Port=7
  wires:
  Silnik elektryczny/1(Obroty) -> Dozownik turbinowy/1(Obroty), Obroty silnika/1
  Dozownik turbinowy/3(Temperatura lozyska) -> Temperatura lozyska/1
  Silnik elektryczny/2(Prad) -> Prad silnika/1
  Dozownik turbinowy/1(Przeplyw) -> Przeplyw/1
  Zalaczenie silnika/1 -> Silnik elektryczny/1(Zalaczenie)
  Poziom zasobnika/1 -> Dozownik turbinowy/2(Poziom zasobnika)
  Zanieczyszczenie lopatek/1 -> Dozownik turbinowy/3(Zanieczyszczenie lopatek)
  "Poslizg przekladni "/1 -> Dozownik turbinowy/5(Poslizg przekladni)
  Uszkodzenie lozyska/1 -> Dozownik turbinowy/7(Uszkodzenie lozyska)
  Dozownik turbinowy/2(Obciazenie silnika) -> Silnik elektryczny/3(Obciazenie zew)
  Wyplnienie komory/1 -> Dozownik turbinowy/6(Wypelnienie komory)
  "Zadane obroty silnika "/1 -> Silnik elektryczny/2(Zadane obroty)
  Uszkodzenie silnika/1 -> Silnik elektryczny/4(Uszkodzenie)
  Blokada przeplywu/1 -> Dozownik turbinowy/4(Blokada przeplywu)
  Silnik elektryczny/3(Idle) -> Silnik Idle/1
  Silnik elektryczny/4(Running) -> Silnik Running/1
  Silnik elektryczny/5(Alarm) -> Silnik Alarm/1
  Przeciek w dozowniku/1 -> Dozownik turbinowy/8(Przeciek w dozowniku)

== system BrowarModel/Mlyn browarniany/Mlyn browarniany/Walce mlyna ==
  note: Walce mlyna + silnik elektryczny
  Zalaczenie silnika : Inport
  "Zadane obroty silnika " : Inport  Port=2
  Doplyw do komory : Inport  Port=3
  Zanieczyszczenie walcow : Inport  Port=4
  Blokada przeplywu : Inport  Port=5
  Przeciek materialu przez walce : Inport  Port=6
  Poslizg przekladni : Inport  Port=7
  Uszkodzenie lozyska : Inport  Port=8
  Uszkodzenie silnika : Inport  Port=9
  Dead Zone : DeadZone  LowerValue=-inf  UpperValue=0.0001
  Komora nad walcami : Subsystem
  Silnik elektryczny : Subsystem
  Walce : Subsystem
  Przeplyw : Outport
  Wypelnienie : Outport  Port=2
  Obroty silnika : Outport  Port=3
  Prad silnika : Outport  Port=4
  Silnik Idle : Outport  Port=5
  Silnik Running : Outport  Port=6
  Silnik Alarm : Outport  Port=7
  Komora nad walcami poziom HI : Outport  Port=8
  Komora nad walcami poziom LO : Outport  Port=9
  Temperatura lozyska : Outport  Port=10
  wires:
  Komora nad walcami/1(Stopien wypelnienie) -> Wypelnienie/1, Walce/2(Wypelnienie komory)
  Silnik elektryczny/1(Obroty) -> Obroty silnika/1, Walce/1(Obroty)
  Walce/1(Przeplyw) -> Komora nad walcami/2(Odplyw), Dead Zone/1
  Walce/2(Obciazenie silnika) -> Silnik elektryczny/3(Obciazenie zew)
  Doplyw do komory/1 -> Komora nad walcami/1(Doplyw)
  Zalaczenie silnika/1 -> Silnik elektryczny/1(Zalaczenie)
  "Zadane obroty silnika "/1 -> Silnik elektryczny/2(Zadane obroty)
  Uszkodzenie silnika/1 -> Silnik elektryczny/4(Uszkodzenie)
  Silnik elektryczny/2(Prad) -> Prad silnika/1
  Komora nad walcami/2(Poziom HI) -> Komora nad walcami poziom HI/1
  Komora nad walcami/3(Poziom LO) -> Komora nad walcami poziom LO/1
  Walce/3(Temperatura lozyska) -> Temperatura lozyska/1
  Zanieczyszczenie walcow/1 -> Walce/3(Zanieczyszczenie walcow)
  Blokada przeplywu/1 -> Walce/4(Blokada przeplywu)
  Poslizg przekladni/1 -> Walce/6(Poslizg przekladni)
  Uszkodzenie lozyska/1 -> Walce/7(Uszkodzenie lozyska)
  Silnik elektryczny/3(Idle) -> Silnik Idle/1
  Silnik elektryczny/4(Running) -> Silnik Running/1
  Silnik elektryczny/5(Alarm) -> Silnik Alarm/1
  Przeciek materialu przez walce/1 -> Walce/5(Przeciek materialu przez walce)
  Dead Zone/1 -> Przeplyw/1

== system BrowarModel/Mlyn browarniany/Mlyn browarniany/Zasobnik dozownika slodu ==
  note: Zasobnik dozownika slodu
  note: Uszkodzenie:
      | Wyciek zewnetrzny w dolnej czesci
      | zasobnika slodu
  Doplyw : Inport
  Odplyw : Inport  Port=2
  Wyciek : Inport  Port=3
  Char. zbiornika : Lookup  InputValues="[0\t0.001\t0.003\t0.010\t0.023\t0.046\t0.079\t0.125\t0.186\t0.264\t0.362\t0.480\t0.622\t0.790\t0.985\t1.210\t1.466\t1.708\t2.008\t2.308\t2.608\t2.908\t3.208\t3.508\t3.808\t4.108\t4.408\t4.708\t5.008\t5.308\t5.608\t5.908\t6.208\t6.508\t6.808\t7.108\t7.408\t7.708\t8.008\t8.308\t8.608\t8.908\t9.208\t9.508\t9.808\t10.108\t10.408\t10.708\t11.008\t11.308\t11.608\t11.908\t12.208\t12.508\t12.808\t13.108\t13.408]"  Table="[0\t0\t0.1\t0.2\t0.3\t0.4\t0.5\t0.6\t0.7\t0.8\t0.9\t1\t1.1\t1.2\t1.3\t1.4\t1.5\t1.6\t1.7\t1.8\t1.9\t2\t2.1\t2.2\t2.3\t2.4\t2.5\t2.6\t2.7\t2.8\t2.9\t3\t3.1\t3.2\t3.3\t3.4\t3.5\t3.6\t3.7\t3.8\t3.9\t4\t4.1\t4.2\t4.3\t4.4\t4.5\t4.6\t4.7\t4.8\t4.9\t5\t5.1\t5.2\t5.3\t5.4\t5.5]"  SaturateOnIntegerOverflow=off
  Detektory poziomu : Subsystem
  Gain : Gain  Gain=1/100
  Integrator (max = 13,69m3) : Integrator  LimitOutput=on  UpperSaturationLimit=13.69  LowerSaturationLimit=0
  Max wyciek : Gain  Gain=0.02
  Product : Product  RndMeth=Zero
  Sat doplyw (F>=0) : Saturate  UpperLimit=inf  LowerLimit=0
  Sat odplyw (F>=0) : Saturate  UpperLimit=inf  LowerLimit=0
  Sat wyciek (0-100) : Saturate  UpperLimit=100  LowerLimit=0
  Sum : Sum  Inputs=|+-
  Sum1 : Sum  Inputs=|+-
  Wyciek char : Lookup  InputValues=[0, 0.5, 0.6, 1]  Table=[0, 0, 1, 1]  SaturateOnIntegerOverflow=off
  Poziom : Outport
  Poziom HI : Outport  Port=2
  Poziom LO : Outport  Port=3
  wires:
  Doplyw/1 -> Sat doplyw (F>=0)/1  "m3/s"
  Odplyw/1 -> Sat odplyw (F>=0)/1  "m3/s"
  Integrator (max = 13,69m3)/1 -> Char. zbiornika/1  "m3"
  Char. zbiornika/1 -> Detektory poziomu/1(Poziom), Wyciek char/1, Poziom/1  "m"
  Sat doplyw (F>=0)/1 -> Sum/1
  Sat odplyw (F>=0)/1 -> Sum/2
  Sum1/1 -> Integrator (max = 13,69m3)/1
  Sum/1 -> Sum1/1  "m3/s"
  Wyciek/1 -> Sat wyciek (0-100)/1  "[0,100]"
  Product/1 -> Sum1/2  "m3/h"
  Detektory poziomu/2(Poziom niski) -> Poziom LO/1
  Detektory poziomu/1(Poziom  wysoki) -> Poziom HI/1
  Sat wyciek (0-100)/1 -> Gain/1
  Wyciek char/1 -> Max wyciek/1  "[0..1]"
  Max wyciek/1 -> Product/2  "m3/h"
  Gain/1 -> Product/1
